simulink model "Li_ion_OneCell_Model"  (R2022a)
settings: Solver=VariableStepAuto  StartTime=0.0  StopTime=350  RelTol=1e-3
values from neighbouring files (symbols this model uses):
  A_d = sys_d.A    [Lithium_ion_oneCell_Modeling_continuous_Linear.m]    (also in Lithium_ion_oneCell_Modeling_continuous_new.m)
  B_d = sys_d.B    [Lithium_ion_oneCell_Modeling_continuous_Linear.m]    (also in Lithium_ion_oneCell_Modeling_continuous_new.m)
  R0 = 43e-3    (= 0.043)    [Lithium_ion_oneCell_Modeling_continuous_Linear.m]    (also in Lithium_ion_oneCell_Modeling_continuous_new.m)
  X0 = [0.6; 0; 0]    [Lithium_ion_oneCell_Modeling_continuous_Linear.m]    (also in Lithium_ion_oneCell_Modeling_continuous_new.m = [0.6;0;0])
undefined symbols (not defined in the file or in its folder): sigbuilder_block
libraries: simulink x1
settings Model: Creator=Asus  LastModifiedBy=Asus

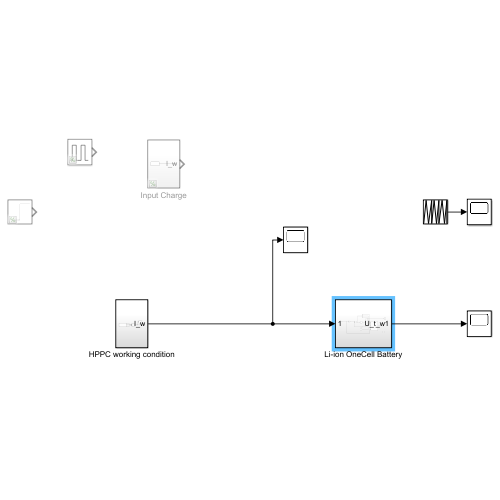
[thumbnail: Simulink's stored preview of the top-level diagram]
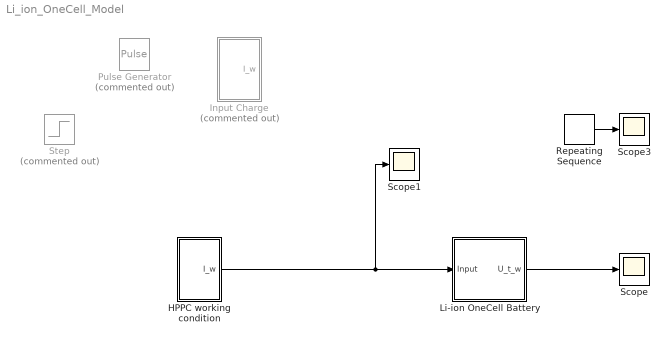
== system Li_ion_OneCell_Model ==
  HPPC working condition : Subsystem
  Input Charge : Subsystem  Commented=on
  Li-ion OneCell Battery : Subsystem
  Pulse Generator : DiscretePulseGenerator  Commented=on  PulseType=Time based  Amplitude=-2.4  Period=0.05  PulseWidth=99
  Repeating Sequence : simulink/Sources/Repeating Sequence  rep_seq_t=[0 2 4 6]  rep_seq_y=[0 10 0 10]
  Scope : Scope
  Scope1 : Scope
  Scope3 : Scope
  Step : Step  Commented=on  Time=90000  Before=-4.8  After=-4.8  SampleTime=0
  wires:
  Li-ion OneCell Battery/1(U_t_w) -> Scope/1
  HPPC working condition/1(I_w) -> Scope1/1, Li-ion OneCell Battery/1(Input)
  Repeating Sequence/1 -> Scope3/1

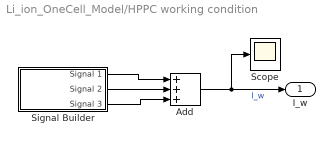
== system Li_ion_OneCell_Model/HPPC working condition ==
  Add : Sum  Inputs=+++
  Scope : Scope
  Signal Builder : Subsystem  Tag=STV Subsys  LoadFcn=sigbuilder_block('load');  StartFcn=sigbuilder_block('start');  StopFcn=sigbuilder_block('stop');  ClipboardFcn=sigbuilder_block('clipboard');  mask(Sigbuilder block){tuvar=[0:10]}
      mask help: Simulink:masks:SigbuilderBlock_MD
      mask init:
      | if ~strcmp(get_param(bdroot(gcbh),'SimulationStatus'),'stopped') tuvar = sigbuilder_block('maskInit'); end
      settings: CopyFcn=sigbuilder_block('copy');  DeleteFcn=sigbuilder_block('delete');  ModelCloseFcn=sigbuilder_block('modelClose');  PreSaveFcn=sigbuilder_block('preSave');  PauseFcn=sigbuilder_block('pause');  ContinueFcn=sigbuilder_block('continue');  NameChangeFcn=sigbuilder_block('namechange');  OpenFcn=sigbuilder_block('open',[5.4 36 1141.2 516.6 ]);  CloseFcn=sigbuilder_block('close');
      mask Display: plot(0, 0, 100, 100,[2, 2, 32, 32, 2], [68, 8, 8, 68, 68],[32, 2], [38, 38], [32, 19, 2],[53, 60, 44], [32, 17, 17, 2],[16, 16, 31, 31]);txt = getActiveGroup(gcbh);text(2, 100, txt,'verticalAlignment', 'top');
  I_w : Outport
  wires:
  Add/1 -> Scope/1, I_w/1  "I_w"
  Signal Builder/2(Signal 2) -> Add/2
  Signal Builder/1(Signal 1) -> Add/1
  Signal Builder/3(Signal 3) -> Add/3

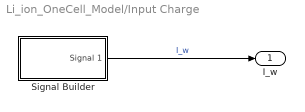
== system Li_ion_OneCell_Model/Input Charge ==
  Signal Builder : Subsystem  Tag=STV Subsys  LoadFcn=sigbuilder_block('load');  StartFcn=sigbuilder_block('start');  StopFcn=sigbuilder_block('stop');  ClipboardFcn=sigbuilder_block('clipboard');  mask(Sigbuilder block){tuvar=[0:10]}
      mask help: Simulink:masks:SigbuilderBlock_MD
      mask init:
      | if ~strcmp(get_param(bdroot(gcbh),'SimulationStatus'),'stopped') tuvar = sigbuilder_block('maskInit'); end
      settings: CopyFcn=sigbuilder_block('copy');  DeleteFcn=sigbuilder_block('delete');  ModelCloseFcn=sigbuilder_block('modelClose');  PreSaveFcn=sigbuilder_block('preSave');  PauseFcn=sigbuilder_block('pause');  ContinueFcn=sigbuilder_block('continue');  NameChangeFcn=sigbuilder_block('namechange');  OpenFcn=sigbuilder_block('open',[5.4 36 1141.2 516.6 ]);  CloseFcn=sigbuilder_block('close');
      mask Display: plot(0, 0, 100, 100,[2, 2, 32, 32, 2], [68, 8, 8, 68, 68],[32, 2], [38, 38], [32, 19, 2],[53, 60, 44], [32, 17, 17, 2],[16, 16, 31, 31]);txt = getActiveGroup(gcbh);text(2, 100, txt,'verticalAlignment', 'top');
  I_w : Outport
  wires:
  Signal Builder/1(Signal 1) -> I_w/1  "I_w"

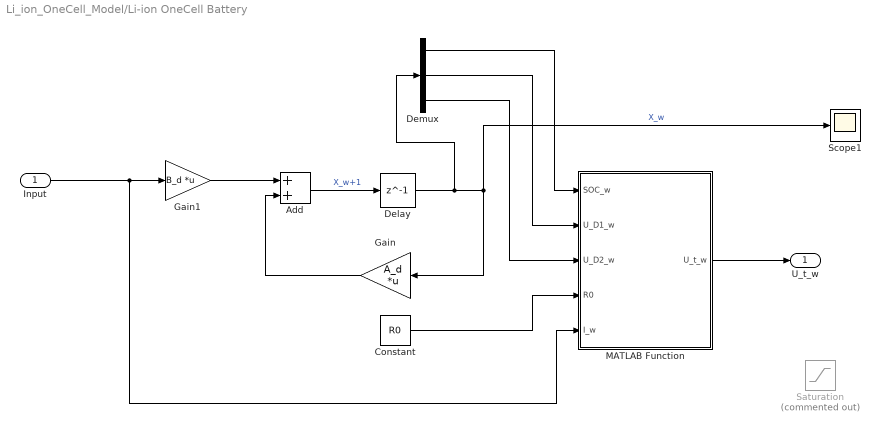
== system Li_ion_OneCell_Model/Li-ion OneCell Battery ==
  Input : Inport
  Add : Sum
  Constant : Constant  Value=R0
  Delay : Delay  DelayLength=1  InitialCondition=X0
  Demux : Demux  Outputs=3
  Gain : Gain  Gain=A_d  Multiplication=Matrix(K*u)
  Gain1 : Gain  Gain=B_d  Multiplication=Matrix(K*u)
  MATLAB Function : MATLAB Function  TreatAsAtomicUnit=on
  Saturation : Saturate  Commented=on  UpperLimit=4.2  LowerLimit=3
  Scope1 : Scope
  U_t_w : Outport
  wires:
  Input/1 -> MATLAB Function/5(I_w), Gain1/1
  Add/1 -> Delay/1  "X_w+1"
  Demux/1 -> MATLAB Function/1(SOC_w)
  Delay/1 -> Demux/1, Gain/1, Scope1/1  "X_w"
  Gain1/1 -> Add/1
  Demux/3 -> MATLAB Function/3(U_D2_w)
  Gain/1 -> Add/2
  Demux/2 -> MATLAB Function/2(U_D1_w)
  Constant/1 -> MATLAB Function/4(R0)
  MATLAB Function/1(U_t_w) -> U_t_w/1

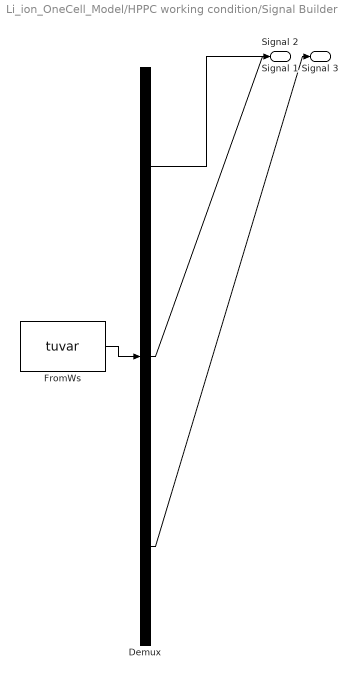
== system Li_ion_OneCell_Model/HPPC working condition/Signal Builder ==
  Demux : Demux  Tag=STV Demux  Outputs=3
      settings: DisplayOption=none
  FromWs : FromWorkspace  Tag=STV FromWs  VariableName=tuvar
      SigBuilderData=|
      | common.afterFinalStr = 'Extrapolate'
      | common.sampleTime = 0
      | dataSet.timeRange = [0 350]
      | dataSet.name = 'Group 1'
      | sbobj.Groups.Name = 'Group 1'
      | sbobj.Groups.Signals(1).Name = 'Signal 1'
      | sbobj.Groups.Signals(1).XData = [0 0.1 1 30 30 350]
      | sbobj.Groups.Signals(1).YData = [0 1 4.8 4.8 0 0]
      | sbobj.Groups.Signals(2).Name = 'Signal 2'
      | sbobj.Groups.Signals(2).XData = [0 70 70 80 80 350]
      | sbobj.Groups.Signals(2).YData = [0 0 -2.4 -2.4 1.2 1.2]
      | sbobj.Groups.Signals(3).Name = 'Signal 3'
      | sbobj.Groups.Signals(3).XData = [0 350]
      | sbobj.Groups.Signals(3).YData = [0 0]
      | sbobj.Groups.TimeRange = [0 350]
  Signal 1 : Outport  Tag=STV Outport
  Signal 2 : Outport  Tag=STV Outport  Port=2
  Signal 3 : Outport  Tag=STV Outport  Port=3
  wires:
  FromWs/1 -> Demux/1
  Demux/1 -> Signal 1/1
  Demux/2 -> Signal 2/1
  Demux/3 -> Signal 3/1

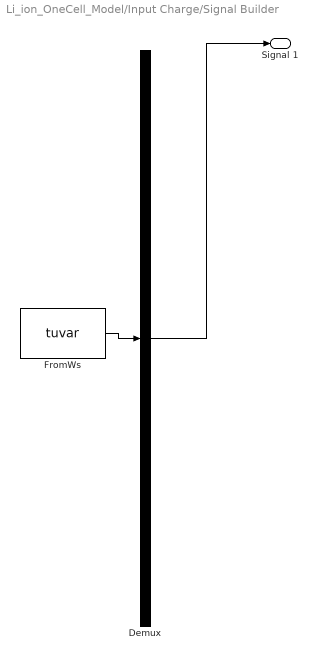
== system Li_ion_OneCell_Model/Input Charge/Signal Builder ==
  Demux : Demux  Tag=STV Demux  Outputs=1
      settings: DisplayOption=none
  FromWs : FromWorkspace  Tag=STV FromWs  VariableName=tuvar
      SigBuilderData=|
      | common.afterFinalStr = 'Extrapolate'
      | common.sampleTime = 0
      | dataSet.timeRange = [0 350]
      | dataSet.name = 'Group 1'
      | sbobj.Groups.Name = 'Group 1'
      | sbobj.Groups.Signals.Name = 'Signal 1'
      | sbobj.Groups.Signals.XData = [0 10 10 200 200 350]
      | sbobj.Groups.Signals.YData = [0 0 -2.4 -2.4 0 0]
      | sbobj.Groups.TimeRange = [0 350]
  Signal 1 : Outport  Tag=STV Outport
  wires:
  FromWs/1 -> Demux/1
  Demux/1 -> Signal 1/1

== matlab function Li_ion_OneCell_Model/Li-ion OneCell Battery/MATLAB Function ==
  data: SOC_w input; U_t_w output; U_D1_w input; U_D2_w input; R0 input; I_w input
function U_t_w = fcn(SOC_w,U_D1_w,U_D2_w,R0,I_w)

p1 = -2744.8612;
p2 = 15237.6802;
p3 = -36711.376;
p4 = 50213.0052;
p5 = -42785.081;
p6 = 23432.4265;
p7 = -8214.5826;
p8 = 1785.199;
p9 = -227.6861;
p10 = 16.3942;
p11 = 3.0665;
f_ocv = p1.*SOC_w.^10 + p2.*SOC_w.^9 + p3.*SOC_w.^8 + p4.*SOC_w.^7 + p5.*SOC_w.^6 + p6.*SOC_w.^5 + p7.*SOC_w.^4 + p8.*SOC_w.^3 + p9.*SOC_w.^2 + p10.*SOC_w + p11;

U_t_w = [0 -1 -1]*[SOC_w;U_D1_w;U_D2_w]-R0*I_w+f_ocv;
